simulink model "iso_calc_temp"  (R2019b)
settings: Solver=VariableStepAuto  StartTime=0.0  StopTime=10.0  RelTol=1e-3
values from neighbouring files (symbols this model uses):
  C = 1    [DataLoop.m]    (also in run_iso_calc.m; testLoop.m = 1.2)
  Tr = 1    [DataLoop.m]    (also in run_iso_calc.m = 0; testLoop.m = 0.38)
  Ts = 1    [DataLoop.m]    (also in run_iso_calc.m = 0; testLoop.m = 0.5)
  Vh = t_current    [run_iso_calc.m]
  Vs = 1    [DataLoop.m]    (also in run_iso_calc.m = -Vh; testLoop.m = 0)
  Zd = 1    [DataLoop.m]    (also in run_iso_calc.m = 0.05; testLoop.m = 0.02)
  Zr = 1    [DataLoop.m]    (also in run_iso_calc.m = 0; testLoop.m = 0)
libraries: ros2lib x1
settings Model: Creator=laiy  LastModifiedBy=laiy

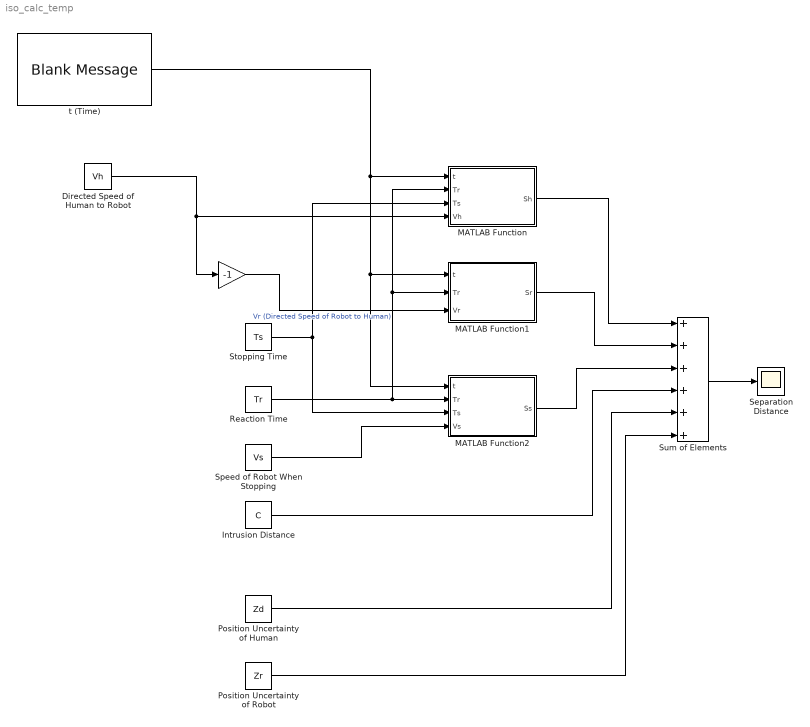
== system iso_calc_temp ==
  " " : Gain  Gain=-1
  Directed Speed of Human to Robot : Constant  Value=Vh
  Intrusion Distance : Constant  Value=C
  MATLAB Function : MATLAB Function  TreatAsAtomicUnit=on
  MATLAB Function1 : MATLAB Function  TreatAsAtomicUnit=on
  MATLAB Function2 : MATLAB Function  TreatAsAtomicUnit=on
  Position Uncertainty of Human : Constant  Value=Zd
  Position Uncertainty of Robot : Constant  Value=Zr
  Reaction Time : Constant  Value=Tr
  Separation Distance : Scope
  Speed of Robot When Stopping : Constant  Value=Vs
  Stopping Time : Constant  Value=Ts
  Sum of Elements : Sum  Inputs=++++++
  t (Time) : ros2lib/Blank Message  messageType=geometry_msgs/Point  SampleTime=inf
      settings: SourceProductName=ROS Toolbox  SourceProductBaseCode=RR
  wires:
  MATLAB Function2/1(Ss) -> Sum of Elements/3
  MATLAB Function/1(Sh) -> Sum of Elements/1
  MATLAB Function1/1(Sr) -> Sum of Elements/2
  Intrusion Distance/1 -> Sum of Elements/4
  Position Uncertainty of Human/1 -> Sum of Elements/5
  Position Uncertainty of Robot/1 -> Sum of Elements/6
  Sum of Elements/1 -> Separation Distance/1
  t (Time)/1 -> MATLAB Function1/1(t), MATLAB Function2/1(t), MATLAB Function/1(t)
  Directed Speed of Human to Robot/1 -> " "/1, MATLAB Function/4(Vh)
  Reaction Time/1 -> MATLAB Function1/2(Tr), MATLAB Function/2(Tr), MATLAB Function2/2(Tr)
  Stopping Time/1 -> MATLAB Function2/3(Ts), MATLAB Function/3(Ts)
  " "/1 -> MATLAB Function1/3(Vr)  "Vr (Directed Speed of Robot to Human)"
  Speed of Robot When Stopping/1 -> MATLAB Function2/4(Vs)

== matlab function iso_calc_temp/MATLAB Function1 ==
  data: t input; Sr output; Tr input; Vr input
function Sr = fcn(t, Tr, Vr)

% Sr = attribute to robot reaction time 
% Vr = max speed of robot

Sr = Vr * Tr;

== matlab function iso_calc_temp/MATLAB Function ==
  data: t input; Sh output; Tr input; Ts input; Vh input
function Sh = fcn(t, Tr, Ts, Vh)

% Sh = change from human location

Sh = Vh;

== matlab function iso_calc_temp/MATLAB Function2 ==
  data: t input; Ss output; Tr input; Ts input; Vs input
function Ss = fcn(t, Tr, Ts, Vs)

% Ss = robot stopping dist
% Assume robot's stopping distance in the directinon 
% that reduces separation distance most.

Ss = Vs;
